simulink model "test1"  (R2019b)
settings: Solver=VariableStepAuto  StartTime=0.0  StopTime=10.0  RelTol=1e-3
settings Model: Creator=ckjh7911t  LastModifiedBy=ckjh7911t

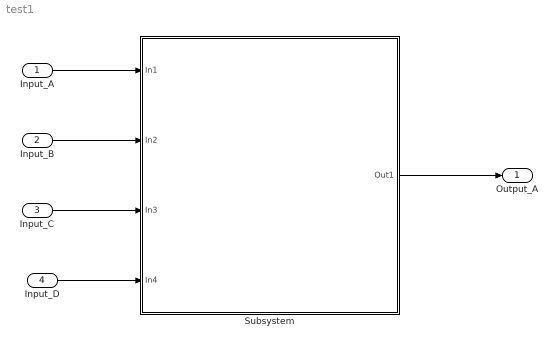
== system test1 ==
  Input_A : Inport
  Input_B : Inport  Port=2
  Input_C : Inport  Port=3
  Input_D : Inport  Port=4
  Subsystem : Subsystem
  Output_A : Outport
  wires:
  Input_C/1 -> Subsystem/3(In3)
  Input_A/1 -> Subsystem/1(In1)
  Input_B/1 -> Subsystem/2(In2)
  Input_D/1 -> Subsystem/4(In4)
  Subsystem/1(Out1) -> Output_A/1

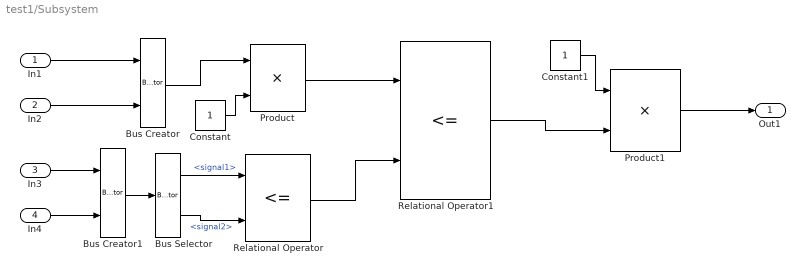
== system test1/Subsystem ==
  In1 : Inport
  In2 : Inport  Port=2
  In3 : Inport  Port=3
  In4 : Inport  Port=4
  Bus Creator : BusCreator  Inputs=2
  Bus Creator1 : BusCreator  Inputs=2
  Bus Selector : BusSelector  OutputSignals=signal1,signal2
  Constant : Constant
  Constant1 : Constant
  Product : Product
  Product1 : Product
  Relational Operator : RelationalOperator  Operator=<=  OutDataTypeStr=boolean  RndMeth=Simplest
  Relational Operator1 : RelationalOperator  Operator=<=  OutDataTypeStr=boolean  RndMeth=Simplest
  Out1 : Outport
  wires:
  In1/1 -> Bus Creator/1
  In2/1 -> Bus Creator/2
  Constant/1 -> Product/2
  Bus Creator/1 -> Product/1
  In3/1 -> Bus Creator1/1
  In4/1 -> Bus Creator1/2
  Bus Creator1/1 -> Bus Selector/1
  Bus Selector/1 -> Relational Operator/1  "<signal1>"
  Bus Selector/2 -> Relational Operator/2  "<signal2>"
  Product/1 -> Relational Operator1/1
  Relational Operator/1 -> Relational Operator1/2
  Relational Operator1/1 -> Product1/2
  Constant1/1 -> Product1/1
  Product1/1 -> Out1/1
